simulink subsystem "Altitude"  (R2024a)
settings: Solver=VariableStepAuto  StartTime=0.0  StopTime=10.0  RelTol=1e-3
undefined symbols (not defined in the file): DiscIntNeverNeededParam, Sim, vehicle
libraries: simulink x1
settings Model: Creator=gurt1  LastModifiedBy=gurt1

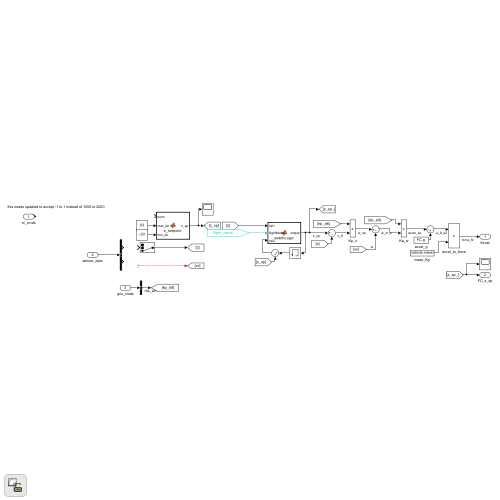
[thumbnail: Simulink's stored preview of the top-level diagram]
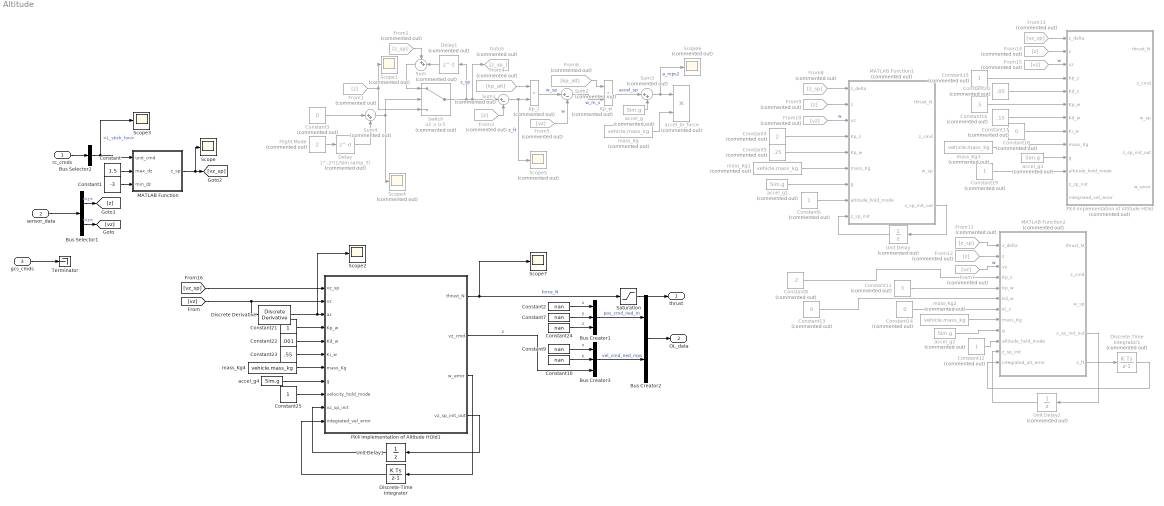
== system Altitude ==
  rc_cmds : Inport
  sensor_data : Inport  Port=2
  gcs_cmds : Inport  Port=3
  Bus Creator1 : BusCreator  Inputs=3
  Bus Creator2 : BusCreator  Inputs=2
  Bus Creator3 : BusCreator  Inputs=3
  Bus Selector1 : BusSelector  OutputSignals=pos_ned_m.z,vel_ned_mps.z
  Bus Selector2 : BusSelector  OutputSignals=sticks.L_stick_lon
  Constant : Constant  Value=1.5
  Constant1 : Constant  Value=-3
  Constant{2,7,9..10,24} (5 alike) : Constant  Value=nan
  Constant11 : Constant  Commented=on  Value=3
  Constant{6,12,15,19} (4 alike) : Constant  Commented=on
  Constant{3,13..14,18} (4 alike) : Constant  Commented=on  Value=0
  Constant16 : Constant  Commented=on  Value=.5
  Constant17 : Constant  Commented=on  Value=.15
  Constant20 : Constant  Commented=on  Value=.05
  Constant21 : Constant
  Constant22 : Constant  Value=.001
  Constant23 : Constant  Value=.55
  Constant25 : Constant
  Constant4 : Constant  Commented=on  Value=2
  Constant5 : Constant  Commented=on  Value=.25
  Constant8 : Constant  Commented=on  Value=.2
  Delay : Delay  Commented=on  DelayLength=2*(1/Sim.samp_T)
  Delay1 : Delay  Commented=on
  Discrete Derivative : simulink/Discrete/Discrete Derivative  gainval=1.0  ICPrevScaledInput=0.0  OutMin=[]  OutMax=[]  OutDataType=fixdt(1, 16)  OutScaling=2^-10  DoSatur=off
  Discrete-Time Integrator : DiscreteIntegrator  SampleTime=-1  ICPrevOutput=DiscIntNeverNeededParam  ICPrevScaledInput=DiscIntNeverNeededParam
  Discrete-Time Integrator1 : DiscreteIntegrator  Commented=on  SampleTime=-1  ICPrevOutput=DiscIntNeverNeededParam  ICPrevScaledInput=DiscIntNeverNeededParam
  Flight Mode : Constant  Commented=on  Value=2
  From{1,3,9,12,14} (5 alike) : From  Commented=on  GotoTag=z
  From{5,7,10,15} (4 alike) : From  Commented=on  GotoTag=vz
  From11 : From  Commented=on  GotoTag=z_sp
  From13 : From  Commented=on  GotoTag=vz_sp
  From2 : From  Commented=on  GotoTag=z_sp
  From4 : From  Commented=on  GotoTag=kp_alt
  From6 : From  Commented=on  GotoTag=kp_alt
  From8 : From  Commented=on  GotoTag=z_sp
  Goto5 : Goto  Commented=on  GotoTag=z_sp_
  Kp_w : Product  Commented=on
  Kp_z : Product  Commented=on
  MATLAB Function : MATLAB Function  TreatAsAtomicUnit=on
  MATLAB Function1 : MATLAB Function  Commented=on  TreatAsAtomicUnit=on
  MATLAB Function2 : MATLAB Function  Commented=on  TreatAsAtomicUnit=on
  PX4 Implementation of Altitude HOld : MATLAB Function  Commented=on  TreatAsAtomicUnit=on
  PX4 Implementation of Altitude HOld1 : MATLAB Function  TreatAsAtomicUnit=on
  Saturation : Saturate  UpperLimit=vehicle.prop.max_T  LowerLimit=0
  Scope{,2..3,7} (4 alike) : Scope
  Scope{1,4..6} (4 alike) : Scope  Commented=on
  Sum : Sum  Commented=on  Inputs=++|
  Sum1 : Sum  Commented=on  Inputs=|+-
  Sum2 : Sum  Commented=on  Inputs=|+-
  Sum3 : Sum  Commented=on  Inputs=|++
  Sum4 : Sum  Commented=on  Inputs=|++
  Switch : Switch  Commented=on  Criteria=u2 > Threshold  Threshold=0.5  SaturateOnIntegerOverflow=off  InputSameDT=off
  Terminator : Terminator
  Unit Delay : UnitDelay  Commented=on  InitialCondition=nan  SampleTime=-1  HasFrameUpgradeWarning=on
  Unit Delay1 : UnitDelay  InitialCondition=nan  SampleTime=-1  HasFrameUpgradeWarning=on
  Unit Delay2 : UnitDelay  Commented=on  InitialCondition=nan  SampleTime=-1  HasFrameUpgradeWarning=on
  accel_g{,1..3} (4 alike) : Constant  Commented=on  Value=Sim.g
  accel_g4 : Constant  Value=Sim.g
  accel_to_force : Product  Commented=on
  mass_Kg{,1..3} (4 alike) : Constant  Commented=on  Value=vehicle.mass_kg
  mass_Kg4 : Constant  Value=vehicle.mass_kg
  thrust : Outport
  OL_data : Outport  Port=2
  wires:
  Constant/1 -> MATLAB Function/2(max_dz)
  Constant1/1 -> MATLAB Function/3(min_dz)
  Switch/1 -> Sum1/1, Goto5/1, Delay1/1  "z_sp"
  Delay1/1 -> Sum/2
  MATLAB Function/1(z_sp) -> Scope/1, [vz_sp]
  From3/1 -> Sum1/2
  Sum1/1 -> Kp_z/2, Scope5/1  "z_ft"
  From4/1 -> Kp_z/1
  Sum2/1 -> Kp_w/2  "w_m_s"
  From6/1 -> Kp_w/1
  accel_g/1 -> Sum3/2
  Sum3/1 -> accel_to_force/1, Scope6/1  "a_mps2"
  PX4 Implementation of Altitude HOld1/1(thrust_N) -> Saturation/1, Scope7/1  "force_N"
  mass_Kg/1 -> accel_to_force/2
  From5/1 -> Sum2/2  "w"
  Kp_z/1 -> Sum2/1  "w_sp"
  Kp_w/1 -> Sum3/1  "accel_sp"
  sensor_data/1 -> Bus Selector1/1
  Bus Selector1/2 -> [vz]  "<z>"
  rc_cmds/1 -> Bus Selector2/1
  Bus Selector2/1 -> MATLAB Function/1(unit_cmd), Scope3/1  "<L_stick_lon>"
  Bus Selector1/1 -> [z]  "<z>"
  gcs_cmds/1 -> Terminator/1
  From1/1 -> Scope1/1, Switch/3
  Flight Mode/1 -> Delay/1
  Delay/1 -> Sum4/2
  Constant3/1 -> Sum4/1
  Sum4/1 -> Scope4/1, Switch/2
  Sum/1 -> Switch/1
  From2/1 -> Sum/1
  Saturation/1 -> thrust/1
  From8/1 -> MATLAB Function1/1(z_delta)
  From9/1 -> MATLAB Function1/2(z)
  From10/1 -> MATLAB Function1/3(vz)  "w"
  Constant4/1 -> MATLAB Function1/4(Kp_z)
  Constant5/1 -> MATLAB Function1/5(Kp_w)
  mass_Kg1/1 -> MATLAB Function1/6(mass_Kg)
  accel_g1/1 -> MATLAB Function1/7(g)
  Constant6/1 -> MATLAB Function1/8(altitude_hold_mode)
  MATLAB Function1/4(z_sp_init_out) -> Unit Delay/1
  Unit Delay/1 -> MATLAB Function1/9(z_sp_init)
  Constant10/1 -> Bus Creator3/2  "y"
  Constant9/1 -> Bus Creator3/1  "x"
  Constant7/1 -> Bus Creator1/2  "y"
  Bus Creator1/1 -> Bus Creator2/1  "pos_cmd_ned_m"
  Bus Creator3/1 -> Bus Creator2/2  "vel_cmd_ned_mps"
  Constant2/1 -> Bus Creator1/1  "x"
  PX4 Implementation of Altitude HOld1/2(vz_cmd) -> Bus Creator3/3  "z"
  Bus Creator2/1 -> OL_data/1
  Unit Delay1/1 -> PX4 Implementation of Altitude HOld1/10(vz_sp_init)
  PX4 Implementation of Altitude HOld1/4(vz_sp_init_out) -> Unit Delay1/1
  Constant12/1 -> MATLAB Function2/10(altitude_hold_mode)
  accel_g2/1 -> MATLAB Function2/9(g)
  mass_Kg2/1 -> MATLAB Function2/8(mass_Kg)
  From7/1 -> MATLAB Function2/3(vz)  "w"
  From12/1 -> MATLAB Function2/2(z)
  From11/1 -> MATLAB Function2/1(z_delta)
  PX4 Implementation of Altitude HOld1/3(w_error) -> Discrete-Time Integrator/1
  Discrete-Time Integrator/1 -> PX4 Implementation of Altitude HOld1/11(integrated_vel_error)
  Constant14/1 -> MATLAB Function2/7(Ki_z)
  Constant8/1 -> MATLAB Function2/4(Kp_z)
  Constant11/1 -> MATLAB Function2/5(Kp_w)
  Constant13/1 -> MATLAB Function2/6(Kd_w)
  From13/1 -> PX4 Implementation of Altitude HOld/1(z_delta)
  From14/1 -> PX4 Implementation of Altitude HOld/2(z)
  From15/1 -> PX4 Implementation of Altitude HOld/3(vz)  "w"
  Constant15/1 -> PX4 Implementation of Altitude HOld/4(Kp_z)
  Constant16/1 -> PX4 Implementation of Altitude HOld/6(Kp_w)
  Constant17/1 -> PX4 Implementation of Altitude HOld/7(Kd_w)
  Constant18/1 -> PX4 Implementation of Altitude HOld/8(Ki_w)
  mass_Kg3/1 -> PX4 Implementation of Altitude HOld/9(mass_Kg)
  accel_g3/1 -> PX4 Implementation of Altitude HOld/10(g)
  Constant19/1 -> PX4 Implementation of Altitude HOld/11(altitude_hold_mode)
  MATLAB Function2/5(z_ft) -> Discrete-Time Integrator1/1
  Discrete-Time Integrator1/1 -> MATLAB Function2/12(integrated_alt_error)
  MATLAB Function2/4(z_sp_init_out) -> Unit Delay2/1
  Unit Delay2/1 -> MATLAB Function2/11(z_sp_init)
  Constant20/1 -> PX4 Implementation of Altitude HOld/5(Kd_z)
  [vz_sp] -> PX4 Implementation of Altitude HOld1/1(vz_sp)
  [vz] -> PX4 Implementation of Altitude HOld1/2(vz), Discrete Derivative/1
  Constant21/1 -> PX4 Implementation of Altitude HOld1/4(Kp_w)
  Constant22/1 -> PX4 Implementation of Altitude HOld1/5(Kd_w)
  Constant23/1 -> PX4 Implementation of Altitude HOld1/6(Ki_w)
  mass_Kg4/1 -> PX4 Implementation of Altitude HOld1/7(mass_Kg)
  accel_g4/1 -> PX4 Implementation of Altitude HOld1/8(g)
  Constant24/1 -> Bus Creator1/3  "z"
  Constant25/1 -> PX4 Implementation of Altitude HOld1/9(velocity_hold_mode)
  Discrete Derivative/1 -> PX4 Implementation of Altitude HOld1/3(az), Scope2/1

== matlab function Altitude/PX4 Implementation of Altitude HOld1 ==
  data: vz_sp input; vz input; az input; Kp_w input; Kd_w input; Ki_w input; mass_Kg input; g input; velocity_hold_mode input; thrust_N output; vz_cmd output; w_error output; vz_sp_init_out output; vz_sp_init input; integrated_vel_error input
%% velocity_controller_px4_style
% DESCRIPTION:
%   This function computes the thrust force required to track a velocity setpoint.
%   It follows the PX4 architecture: A PID velocity controller generates an acceleration setpoint.
%
% INPUTS:
%   vz_sp - Pilot-commanded vertical velocity setpoint (positive down) [m/s]
%   vz - Current vertical velocity (positive down) [m/s]
%   Kp_w - Proportional gain for velocity control [-]
%   Kd_w - Damping gain for velocity control [-]
%   Ki_w - Integral gain for velocity control [-]
%   mass_Kg - Vehicle mass [kg]
%   g - Gravitational acceleration [m/s^2]
%   velocity_hold_mode - Boolean flag for velocity hold (1 = hold, 0 = no hold)
%   vz_sp_init - Previous velocity setpoint (NaN if not set) [m/s]
%   integrated_vel_error - Integrated velocity error from Simulink [m/s]
%
% OUTPUTS:
%   thrust_N - Required thrust force [N]
%   vz_cmd - Locked desired velocity setpoint [m/s]
%   w_error - Velocity error [m/s]
%   vz_sp_init_out - Updated velocity setpoint for future calls [m/s]
%
% WRITTEN BY:
%   Garrett D. Asper
%   Virginia Tech
%   Email: garrettasper@vt.edu
%
% HISTORY:
%   [Date] - Created and debugged, GDA
%
% NOMENCLATURE:                                  UNITS:
%   Not Applicable                                  Not Applicable.

function [thrust_N, vz_cmd, w_error, vz_sp_init_out] = velocity_controller_px4_style(vz_sp, vz, az, Kp_w, Kd_w, Ki_w, mass_Kg, g, velocity_hold_mode, vz_sp_init, integrated_vel_error)

    % Velocity Hold Logic
    % If in velocity hold mode and vz_sp_init has not been set, initialize it
    if velocity_hold_mode == 1 && isnan(vz_sp_init)
        vz_sp_init = vz;  % Lock in the current velocity as the initial setpoint
    end

    % If not in velocity hold mode, reset vz_sp_init to the current velocity
    if velocity_hold_mode == 0
        vz_sp_init = vz;
    end

    % If velocity hold mode is active, use the locked setpoint (vz_sp_init)
    if velocity_hold_mode == 1
        vz_cmd = vz_sp_init + vz_sp;  % Desired velocity is locked + pilot input
    else
        % If not in hold mode, follow the pilot's commands directly
        vz_cmd = vz_sp;
    end

    % Velocity Control Loop (PID Controller)

    % Velocity error (difference between desired and actual vertical speed)
    w_error = vz_cmd - vz;

    % Proportional term for velocity control
    proportional_term = Kp_w * w_error;

    % Integral term for velocity control
    integral_term = Ki_w * integrated_vel_error;

    % Derivative term for velocity control (damping term)
    derivative_term = Kd_w * (az);  % Damping on current velocity

    % Desired acceleration (accel_sp) based on velocity error, proportional, integral, and damping
    accel_sp = proportional_term + integral_term - derivative_term;

    % Net acceleration to be provided by thrust (subtract gravity)
    a_mps2 = -accel_sp + g;

    % Required thrust force
    thrust_N = mass_Kg * a_mps2;

    % Output the updated velocity setpoint (either new value or NaN)
    vz_sp_init_out = vz_sp_init;

end

== matlab function Altitude/MATLAB Function ==
  data: unit_cmd input; z_sp output; max_dz input; min_dz input
function z_sp = z_setpoint(unit_cmd, max_dz, min_dz)
    % Original PWM signal range
    minValue = -1;
    maxValue = 1;

    % Normalize the PWM signal between 0 and 100%
    throttlecmd = ((unit_cmd - minValue) / (maxValue - minValue)) * 100;

    % Define thresholds for mapping
    lowerThreshold = 40;
    upperThreshold = 60;

    % Map values based on thresholds
    if throttlecmd < lowerThreshold
        z_sp = -((lowerThreshold - throttlecmd) / lowerThreshold) * min_dz;
    elseif throttlecmd > upperThreshold
        z_sp = -((throttlecmd - upperThreshold) / (100 - upperThreshold)) * max_dz;
    else
        % Failsafe: Set z_sp to 0 if it's between lowerThreshold and upperThreshold
        z_sp = 0;
    end
end

== matlab function Altitude/MATLAB Function1 ==
  data: z_delta input; thrust_N output; z input; vz input; Kp_z input; Kp_w input; mass_Kg input; g input; z_cmd output; w_sp output; altitude_hold_mode input; z_sp_init input; z_sp_init_out output
%% altitude_controller
% DESCRIPTION:
%   This function computes the thrust force required to track a set altitude.
%   It locks the altitude setpoint (z_cmd) when in altitude hold mode,
%   and updates it only when the pilot commands a change in altitude.
%
% INPUTS:
%   z_delta - Pilot-commanded change in altitude (positive down) [m]
%   z - Current altitude (positive down) [m]
%   vz - Current vertical velocity (positive down) [m/s]
%   Kp_z - Proportional gain for altitude control [-]
%   Kp_w - Proportional gain for vertical speed control [-]
%   mass_Kg - Vehicle mass [kg]
%   g - Gravitational acceleration [m/s^2]
%   altitude_hold_mode - Boolean flag for altitude hold (1 = hold, 0 = no hold)
%   z_sp_init - Previous altitude setpoint (NaN if not set) [m]
%
% OUTPUTS:
%   thrust_N - Required thrust force [N]
%   z_cmd - Locked desired altitude setpoint [m]
%   z_sp_init_out - Updated altitude setpoint for future calls [m]
%
% WRITTEN BY:
%   Garrett D. Asper
%   Virginia Tech
%   Email: garrettasper@vt.edu
%
% HISTORY:
%   [Date] - Created and debugged, GDA
%
% NOMENCLATURE:                                  UNITS:
%   Not Applicable                                  Not Applicable.

function [thrust_N, z_cmd, w_sp, z_sp_init_out ] = altitude_controller(z_delta, z, vz, Kp_z, Kp_w, mass_Kg, g, altitude_hold_mode, z_sp_init)

    % If in altitude hold mode and z_sp_init has not been set, initialize it
    if altitude_hold_mode == 1 && isnan(z_sp_init)
        z_sp_init = z;  % Lock in the current altitude as the initial setpoint
    end

    % If not in altitude hold mode, reset z_sp_init to NaN
    if altitude_hold_mode == 0
        z_sp_init = z;
    end

    % If altitude hold mode is active, use the locked setpoint (z_sp_init)
    if altitude_hold_mode == 1
        z_cmd = z_sp_init + z_delta;  % Desired altitude is locked + pilot input
    else
        % If not in hold mode, follow the pilot's commands directly
        z_cmd = z + z_delta;
    end

    % Altitude error
    z_ft = z_cmd - z;
    
    % Desired vertical speed (w_sp) based on altitude error and Kp_z
    w_sp = Kp_z * z_ft;

    % Velocity error (difference between desired and actual vertical speed)
    w_error = w_sp - vz;

    % Desired acceleration (accel_sp) based on velocity error and Kp_w
    accel_sp = Kp_w * w_error;

    % Net acceleration to be provided by thrust (subtract gravity)
    a_mps2 = -accel_sp + g;

    % Required thrust force
    thrust_N = mass_Kg * a_mps2;

    % Output the updated altitude setpoint (either new value or NaN)
    z_sp_init_out = z_sp_init;

end

== matlab function Altitude/MATLAB Function2 ==
  data: z_delta input; thrust_N output; z input; vz input; Kp_z input; Kp_w input; Kd_w input; Ki_z input; mass_Kg input; g input; z_cmd output; w_sp output; altitude_hold_mode input; z_sp_init input; z_sp_init_out output; integrated_alt_error input; z_ft output
%% altitude_controller_with_integral_and_damping
% DESCRIPTION:
%   This function computes the thrust force required to track a set altitude.
%   It includes a proportional, integral, and damping term for altitude control.
%
% INPUTS:
%   z_delta - Pilot-commanded change in altitude (positive down) [m]
%   z - Current altitude (positive down) [m]
%   vz - Current vertical velocity (positive down) [m/s]
%   Kp_z - Proportional gain for altitude control [-]
%   Kp_w - Proportional gain for vertical speed control [-]
%   Kd_w - Damping gain for velocity control [-]
%   Ki_z - Integral gain for altitude control [-]
%   mass_Kg - Vehicle mass [kg]
%   g - Gravitational acceleration [m/s^2]
%   altitude_hold_mode - Boolean flag for altitude hold (1 = hold, 0 = no hold)
%   z_sp_init - Previous altitude setpoint (NaN if not set) [m]
%   integrated_alt_error - Integrated altitude error from Simulink [m*s]
%
% OUTPUTS:
%   thrust_N - Required thrust force [N]
%   z_cmd - Locked desired altitude setpoint [m]
%   w_sp - Desired vertical speed [m/s]
%   z_sp_init_out - Updated altitude setpoint for future calls [m]
%
% WRITTEN BY:
%   Garrett D. Asper
%   Virginia Tech
%   Email: garrettasper@vt.edu
%
% HISTORY:
%   [Date] - Created and debugged, GDA
%
% NOMENCLATURE:                                  UNITS:
%   Not Applicable                                  Not Applicable.

function [thrust_N, z_cmd, w_sp, z_sp_init_out,z_ft] = altitude_controller_with_integral_and_damping(z_delta, z, vz, Kp_z, Kp_w, Kd_w, Ki_z, mass_Kg, g, altitude_hold_mode, z_sp_init, integrated_alt_error)

    % If in altitude hold mode and z_sp_init has not been set, initialize it
    if altitude_hold_mode == 1 && isnan(z_sp_init)
        z_sp_init = z;  % Lock in the current altitude as the initial setpoint
    end

    % If not in altitude hold mode, reset z_sp_init to NaN
    if altitude_hold_mode == 0
        z_sp_init = z;
    end

    % If altitude hold mode is active, use the locked setpoint (z_sp_init)
    if altitude_hold_mode == 1
        z_cmd = z_sp_init + z_delta;  % Desired altitude is locked + pilot input
    else
        % If not in hold mode, follow the pilot's commands directly
        z_cmd = z + z_delta;
    end

    % Altitude error
    z_ft = z_cmd - z;
    
    % Desired vertical speed (w_sp) based on altitude error and Kp_z
    w_sp = Kp_z * z_ft;

    % Velocity error (difference between desired and actual vertical speed)
    w_error = w_sp - vz;

    % Integral correction term based on altitude error
    integral_term = Ki_z * integrated_alt_error;

    % Desired acceleration (accel_sp) based on velocity error, Kp_w, damping gain, and integral term
    accel_sp = Kp_w * w_error - Kd_w * vz + integral_term;  % Integral term added

    % Net acceleration to be provided by thrust (subtract gravity)
    a_mps2 = -accel_sp + g;

    % Required thrust force
    thrust_N = mass_Kg * a_mps2;

    % Output the updated altitude setpoint (either new value or NaN)
    z_sp_init_out = z_sp_init;

end

== matlab function Altitude/PX4 Implementation of Altitude HOld ==
  data: z_delta input; thrust_N output; z input; vz input; Kp_z input; Kd_z input; Kp_w input; Kd_w input; Ki_w input; mass_Kg input; g input; z_cmd output; w_sp output; altitude_hold_mode input; z_sp_init input; z_sp_init_out output; integrated_vel_error input; w_error output
%% altitude_controller_px4_style
% DESCRIPTION:
%   This function computes the thrust force required to track a set altitude.
%   It follows the PX4 architecture: A proportional position controller generates
%   a velocity setpoint, and a PID velocity controller generates an acceleration setpoint.
%
% INPUTS:
%   z_delta - Pilot-commanded change in altitude (positive down) [m]
%   z - Current altitude (positive down) [m]
%   vz - Current vertical velocity (positive down) [m/s]
%   Kp_z - Proportional gain for altitude control [-]
%   Kp_w - Proportional gain for velocity control [-]
%   Kd_w - Damping gain for velocity control [-]
%   Ki_w - Integral gain for velocity control [-] (Note: Changed from altitude)
%   mass_Kg - Vehicle mass [kg]
%   g - Gravitational acceleration [m/s^2]
%   altitude_hold_mode - Boolean flag for altitude hold (1 = hold, 0 = no hold)
%   z_sp_init - Previous altitude setpoint (NaN if not set) [m]
%   integrated_vel_error - Integrated velocity error from Simulink [m/s]
%
% OUTPUTS:
%   thrust_N - Required thrust force [N]
%   z_cmd - Locked desired altitude setpoint [m]
%   w_sp - Desired vertical speed [m/s]
%   z_sp_init_out - Updated altitude setpoint for future calls [m]
%   z_ft - Altitude error [m]
%
% WRITTEN BY:
%   Garrett D. Asper
%   Virginia Tech
%   Email: garrettasper@vt.edu
%
% HISTORY:
%   [Date] - Created and debugged, GDA
%
% NOMENCLATURE:                                  UNITS:
%   Not Applicable                                  Not Applicable.

function [thrust_N, z_cmd, w_sp, z_sp_init_out, w_error] = altitude_controller_px4_style(z_delta, z, vz, Kp_z, Kd_z, Kp_w, Kd_w, Ki_w, mass_Kg, g, altitude_hold_mode, z_sp_init, integrated_vel_error)

    % Position Control Loop (P Controller)
    
    % If in altitude hold mode and z_sp_init has not been set, initialize it
    if altitude_hold_mode == 1 && isnan(z_sp_init)
        z_sp_init = z;  % Lock in the current altitude as the initial setpoint
    end

    % If not in altitude hold mode, reset z_sp_init to current altitude
    if altitude_hold_mode == 0
        z_sp_init = z;
    end

    % If altitude hold mode is active, use the locked setpoint (z_sp_init)
    if altitude_hold_mode == 1
        z_cmd = z_sp_init + z_delta;  % Desired altitude is locked + pilot input
    else
        % If not in hold mode, follow the pilot's commands directly
        z_cmd = z + z_delta;
    end

    % Altitude error
    z_ft = z_cmd - z;

    % Derivative term
    derivative_term_z = Kd_z * z;

    % Proportional position controller generates the velocity setpoint (w_sp)
    w_sp = Kp_z * z_ft - derivative_term_z;  % Velocity setpoint generated from position error

    % Velocity Control Loop (PID Controller)

    % Velocity error (difference between desired and actual vertical speed)
    w_error = w_sp - vz;

    % Integral term for velocity control
    integral_term = Ki_w * integrated_vel_error;

    % Derivative term for velocity control (damping term)
    derivative_term = Kd_w * (vz);  % Damping on current velocity

    % Desired acceleration (accel_sp) based on velocity error, proportional, integral, and damping
    accel_sp = Kp_w * w_error + integral_term - derivative_term;

    % Net acceleration to be provided by thrust (subtract gravity)
    a_mps2 = -accel_sp + g;

    % Required thrust force
    thrust_N = mass_Kg * a_mps2;

    % Output the updated altitude setpoint (either new value or NaN)
    z_sp_init_out = z_sp_init;

end
